simulink model "labwrk"  (Simulink 2.09)
settings: Solver=ode45  StartTime=0.0  StopTime=20.0  RelTol=1e-3  AbsTol=1e-6
settings Model: ConsistencyChecking=off  RTWTemplateMakefile=grt_vc.tmf

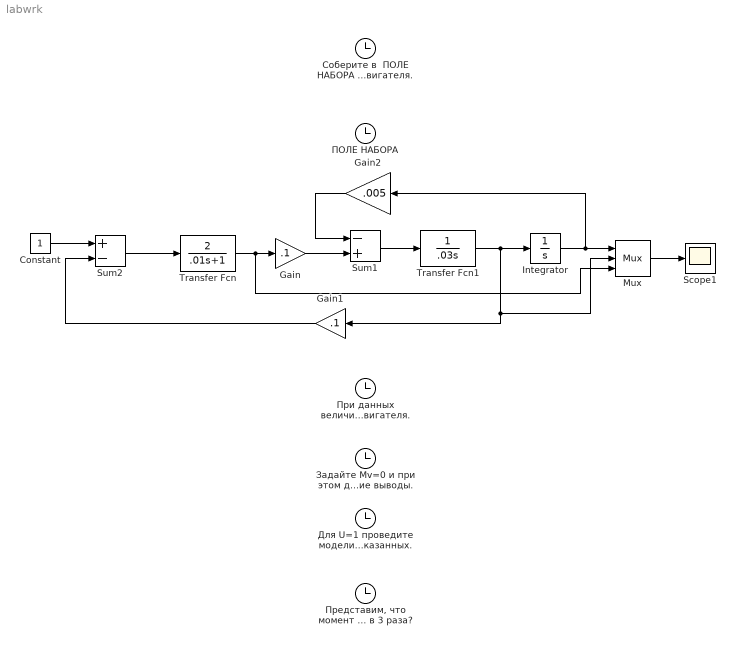
== system labwrk ==
  Constant : Constant  Value=1
  Gain : Gain  Gain=.1
  Gain1 : Gain  Orientation=left  Gain=.1
  Gain2 : Gain  Orientation=left  Gain=.005
  Integrator : Integrator  ExternalReset=none  InitialConditionSource=internal  InitialCondition=0  LimitOutput=off  UpperSaturationLimit=inf  LowerSaturationLimit=-inf  ShowSaturationPort=off  ShowStatePort=off  AbsoluteTolerance=auto
  Mux : Mux  Inputs=3
  Scope1 : Scope
      settings: TickLabels=on  TimeRange=auto  YMin=-5  YMax=50  SaveToWorkspace=off  SaveName=ScopeData
  Sum1 : Sum  Inputs=-+
  Sum2 : Sum  Inputs=+-
  Transfer Fcn : TransferFcn  Numerator=2  Denominator=[.01 1]
  Transfer Fcn1 : TransferFcn  Numerator=[1]  Denominator=[.03 0]
  "Для U=1 проведите моделирование переходного процесса по скорости вала двигателя для значений J=0.05; 0.1; 0.15. Сделайте вывод о  влиянии момента инерции вала на скоростные качества двигателя.  Сделайте вывод,  \"насколько\"  медленнее вращается вал двигателя при  увеличении момента инерции (по осциллограммам угла поворота вала дв.). Если необходимо,дополнительно задайте значения J выше указанных." : Clock
  Задайте Mv=0 и при этом для значений U=0.5; 1.5;  2 получите и зарисуйте осциллограммы скорости и угла вала двигателя. Сделайте над- лежащие выводы. : Clock
  ПОЛЕ НАБОРА : Clock
  "Представим, что момент внешних сил пропорционален с коэффициентом к=0.005: 1) скорости вращения вала дв.; 2) углу поворота вала. Иссле- дуйте моделированием влияние таких связей на переходные процессы двигателя по скорости и повороту для U=1, J=0.03. Ответьте на вопрос: как изменятся эти процессы, если коэффициент пропорциональности  внешнего момента увеличить в 3 раза?" : Clock
  "При данных величинах напряжения на якорной обмотке U и внешнего момента Mv получите и зарисуйте в отчет осциллограммы координат тока, скорости и угла поворота вала двигателя. Затем получите аналогичные осциллограммы при значениях Mv =0 и Mv = 0.15.  Сделайте соответствующий вывод о влиянии момента внешних сил на характер переходного процесса вращения вала двигателя." : Clock
  "Соберите в  ПОЛЕ НАБОРА  вторую модель, используя следующие численные значения: U=1,  Mv=0.05, T=0.01, K=0.1, k=0.1, J=0.01. Подключите виртуальные осциллографы: 1) к выходной координате вала двигателя (углу поворота) 2) через смеситель Mux к координатам тока и скорости двигателя." : Clock
  wires:
  Transfer Fcn/1 -> Mux/3, Gain/1
  Constant/1 -> Sum2/1
  Sum2/1 -> Transfer Fcn/1
  Gain/1 -> Sum1/2
  Sum1/1 -> Transfer Fcn1/1
  Gain1/1 -> Sum2/2
  Transfer Fcn1/1 -> Gain1/1, Mux/2, Integrator/1
  Gain2/1 -> Sum1/1
  Mux/1 -> Scope1/1
  Integrator/1 -> Mux/1, Gain2/1
